simulink model "wcdma_phlayer"  (Simulink 6.0)
settings: Solver=FixedStepDiscrete  SolverMode=SingleTasking  StartTime=0.0  StopTime=0.1  RelTol=1e-3
PreLoadFcn:
  | wcdma_loadinitphlayer;
model workspace: external: M-Code (data not in the file)
undefined symbols (not defined in the file or in its folder): AWGN, Fs, Multipath, slcm, totalBitsDelay, trBlkSetSize, tti
libraries: wcdma_lib x8, dspbuff3 x6, commsink2 x5, dspsnks4 x4, commrandsrc2 x2, commsequence2 x1, dspsigattribs x1, dspsrcs4 x1
CloseFcn:
  | % Clear coding settings
  | clear trBlkSetSize trBlkSize numTrBlks crcSize tti errorCorrMask errorCorr numBitsRF numBitsRM numPhCH posTrCh RMAttribute totalBitsDelay
  | 
  | % Clear antenna settings
  | clear pilotBits overSampling slotFormat sprdFactor scrCode dpchCode numTapsChEst numTapsRRC enableMultipath propConditions
  | 
  | % Clear channel settings
  | clear dopplerFreq snrdB fingerEnables fingerPhases fingerPhasesTicks powerVector fingerPowers
  | 
  | % Clear logging signal
  | clear wcdmaSigsOut
settings Model: Creator=arodrigu  LastModifiedBy=arodrigu  ExtModeAutoUpdateStatusClock=off  ProdHWDeviceType=Specified
settings DataIOCC: LimitDataPoints=off  SaveOutput=off  SaveTime=off  SignalLoggingName=wcdmaSigsOut
settings OptimizationCC: BooleanDataType=off  InlineParams=on
settings DebuggingCC: CheckExecutionContextPreStartOutputMsg=on  CheckExecutionContextRuntimeOutputMsg=on  SolverPrmCheckMsg=none  InheritedTsInSrcMsg=none
settings HardwareCC: ProdHWDeviceType=Specified
settings ModelReferenceCC: UpdateModelReferenceTargets=IfOutOfDate
settings CodeAppCC: MangleLength=5

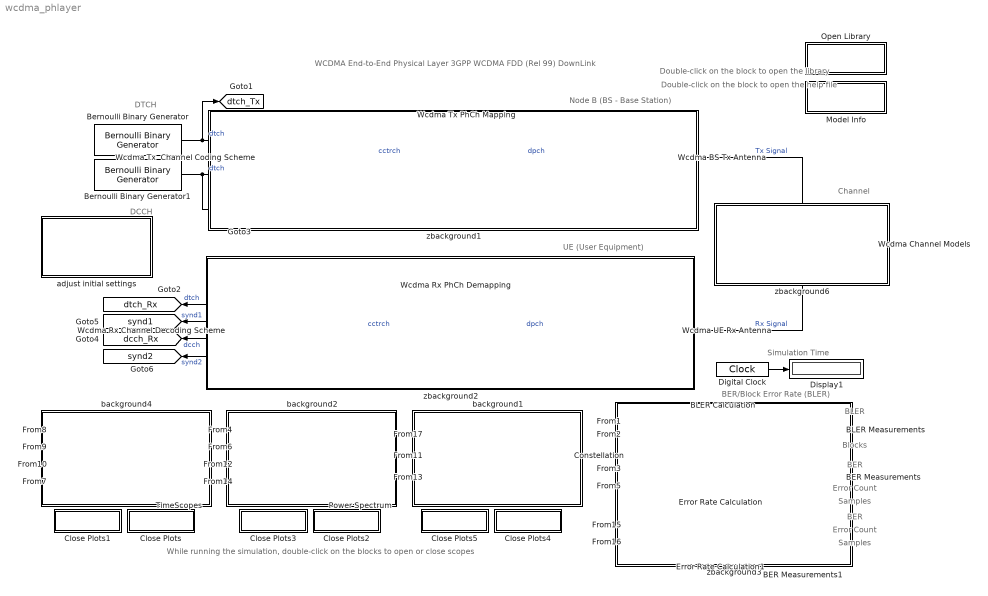
== system wcdma_phlayer ==
  note: DTCH
  note: DCCH
  note: BER
  note: Error Count
  note: Samples
  note: BER/Block Error Rate (BLER)
  note: BLER
  note: Node B (BS - Base Station)
  note: UE (User Equipment)
  note: Channel
  note: WCDMA End-to-End Physical Layer
      | 3GPP WCDMA FDD (Rel 99) DownLink
  note: Blocks
  note: Simulation Time
  note: BER
  note: Error Count
  note: Samples
  note: Double-click on the block
      | to open the help file
  note: While running the simulation, double-click on the blocks to open or close scopes
  note: Double-click on the block
      | to open the library
  BER Measurements : Display
  BER Measurements1 : Display
  BLER Calculation : wcdma_lib/Wcdma Common/BLER Calculation  trBlkSetSize=trBlkSetSize  tti=tti  numBitsDelay=totalBitsDelay
  BLER Measurements : Display
  Bernoulli Binary Generator : commrandsrc2/Bernoulli Binary Generator  P=0.5  seed=[123456]  Ts=(tti(1)*1e-3)/trBlkSetSize(1)  frameBased=on  sampPerFrame=trBlkSetSize(1)  orient=off
  Bernoulli Binary Generator1 : commrandsrc2/Bernoulli Binary Generator  P=0.5  seed=[123456]  Ts=(tti(2)*1e-3)/trBlkSetSize(2)  frameBased=on  sampPerFrame=trBlkSetSize(2)  orient=off
  Close Plots : Subsystem  PropExecContextAcrossSSBoundary=on
      settings: OpenFcn=|
      | ssName = gcs;
      |   set_param([ssName '/TimeScopes/Real Part'],'Open','off');
      |   set_param([ssName '/TimeScopes/Imag Part'],'Open','off');
      |   set_param([ssName '/TimeScopes/Channel Estimates'],'Open','off');
      mask Display: disp('Close Scopes');
  Close Plots1 : Subsystem  PropExecContextAcrossSSBoundary=on
      settings: OpenFcn=|
      | ssName=gcs;
      | set_param([ssName '/TimeScopes/Real Part'],'Open','on');
      |   set_param([ssName '/TimeScopes/Imag Part'],'Open','on');
      |   set_param([ssName '/TimeScopes/Channel Estimates'],'Open','on');
      mask Display: disp('Open Scopes');
  Close Plots2 : Subsystem  PropExecContextAcrossSSBoundary=on
      settings: OpenFcn=|
      | set_param([gcs '/Power Spectrum/Before Spreading Spectrum'],'OpenScopeAtSimStart','off');
      |   set_param([gcs '/Power Spectrum/Before Pulse Shaping'],'OpenScopeAtSimStart','off');
      |   set_param([gcs '/Power Spectrum/Tx Signal'],'OpenScopeAtSimStart','off');
      |   set_param([gcs '/Power Spectrum/Rx Signal'],'OpenScopeAtSimStart','off');
      |   sdspfscope2([],[],[],'ScopeUpdate',[gcs '/Power Spectrum/Before Spreading Spectrum'],'CloseFig');
      |   sdspfscope2([],[],[],'ScopeUpdate',[gcs '/Power Spectrum/Before Pulse Shaping'],'CloseFig');
      |   sdspfscope2([],[],[],'ScopeUpdate',[gcs '/Power Spectrum/Tx Signal'],'CloseFig');
      |   sdspfscope2([],[],[],'ScopeUpdate',[gcs '/Power Spectrum/Rx Signal'],'CloseFig');
      mask Display: disp('Close Scopes');
  Close Plots3 : Subsystem  PropExecContextAcrossSSBoundary=on
      settings: OpenFcn=|
      | set_param([gcs '/Power Spectrum/Before Spreading Spectrum'],'OpenScopeAtSimStart','on');
      |   set_param([gcs '/Power Spectrum/Before Pulse Shaping'],'OpenScopeAtSimStart','on');
      |   set_param([gcs '/Power Spectrum/Tx Signal'],'OpenScopeAtSimStart','on');
      |   set_param([gcs '/Power Spectrum/Rx Signal'],'OpenScopeAtSimStart','on');
      |   sdspfscope2([],[],[],'ScopeUpdate',[gcs '/Power Spectrum/Before Spreading Spectrum'],'OpenFig');
      |   sdspfscope2([],[],[],'ScopeUpdate',[gcs '/Power Spectrum/Before Pulse Shaping'],'OpenFig');
      |   sdspfscope2([],[],[],'ScopeUpdate',[gcs '/Power Spectrum/Tx Signal'],'OpenFig');
      |   sdspfscope2([],[],[],'ScopeUpdate',[gcs '/Power Spectrum/Rx Signal'],'OpenFig');
      mask Display: disp('Open Scopes');
  Close Plots4 : Subsystem  PropExecContextAcrossSSBoundary=on
      settings: OpenFcn=|
      | set_param([bdroot '/Constellation/DPCH_Rx'],'OpenScopeAtSimStart','off');
      | set_param([bdroot '/Constellation/DPCH_Derot'],'OpenScopeAtSimStart','off');
      | set_param([bdroot '/Constellation/DPCH_Comb'],'OpenScopeAtSimStart','off');
      | sdspfscope2([],[],[],'ScopeUpdate',[bdroot '/Constellation/DPCH_Rx'],'CloseFig');
      | sdspfscope2([],[],[],'ScopeUpdate',[bdroot '/Constellation/DPCH_Derot'],'CloseFig');
      | sdspfscope2([],[],[],'ScopeUpdate',[bdroot '/Constellation/DPCH_Comb'],'CloseFig');
      mask Display: disp('Close Scopes');
  Close Plots5 : Subsystem  PropExecContextAcrossSSBoundary=on
      settings: OpenFcn=|
      | sdspfscope2([],[],[],'ScopeUpdate',[bdroot '/Constellation/DPCH_Rx'],'OpenFig');
      | sdspfscope2([],[],[],'ScopeUpdate',[bdroot '/Constellation/DPCH_Derot'],'OpenFig');
      | sdspfscope2([],[],[],'ScopeUpdate',[bdroot '/Constellation/DPCH_Comb'],'OpenFig');
      | set_param([bdroot '/Constellation/DPCH_Rx'],'OpenScopeAtSimStart','on');
      | set_param([bdroot '/Constellation/DPCH_Derot'],'OpenScopeAtSimStart','on');
      | set_param([bdroot '/Constellation/DPCH_Comb'],'OpenScopeAtSimStart','on');
      mask Display: disp('Open Scopes');
  Constellation : Subsystem  TreatAsAtomicUnit=on  PropExecContextAcrossSSBoundary=on
      mask Display: disp('Scatter\nPlot')
  Digital Clock : DigitalClock  SampleTime=0.001
  Display1 : Display
  Error Rate Calculation : commsink2/Error Rate Calculation  N=totalBitsDelay(1)  st_delay=0  cp_mode=Entire frame  subframe=[]  PMode=Port  WsName=ErrorVec  RsMode2=off  stop=off  numErr=100  maxBits=1e6
  Error Rate Calculation1 : commsink2/Error Rate Calculation  N=totalBitsDelay(2)  st_delay=0  cp_mode=Entire frame  subframe=[]  PMode=Port  WsName=ErrorVec  RsMode2=off  stop=off  numErr=100  maxBits=1e6
  Model Info : Subsystem  LoadFcn=slcm LoadBlock;  InitFcn=slcm('UpdateAllCMBlocksInThisModelInit')  PropExecContextAcrossSSBoundary=on  mask(CMBlock){InitialSaveTempField=, InitialBlockCM=none, BlockCM=none, Frame=on, SaveTempField=, DisplayStringWithTags=Info, MaskDisplayString=Info, HorizontalTextAlignment=Center, LeftAlignmentValue=0.5, SourceBlockDiagram=wcdma_phlayer, TagMaxNumber=20, CMTag1=, CMTag2=, CMTag3=, CMTag4=, CMTag5=, CMTag6=, CMTag7=, CMTag8=, CMTag9=, CMTag10=, CMTag11=, CMTag12=, CMTag13=, CMTag14=, CMTag15=, CMTag16=, CMTag17=, CMTag18=, CMTag19=, CMTag20=}
      mask help: This block allows revision control information to be displayed within the model.
      settings: CopyFcn=slcm CopyBlock;  DeleteFcn=slcm Cancel;  PostSaveFcn=slcm('UpdateAllCMBlocksInThisModel')  NameChangeFcn=slcm Rename;  OpenFcn=commdemohelp;
      mask Display: text(str2num(LeftAlignmentValue), 0.5, MaskDisplayString, 'HorizontalAlignment', HorizontalTextAlignment)
  Open Library : Subsystem  PropExecContextAcrossSSBoundary=on
      settings: OpenFcn=open('wcdma_lib.mdl');
      mask Display: disp('WCDMA\nLibrary')
  Power Spectrum : Subsystem  TreatAsAtomicUnit=on  PropExecContextAcrossSSBoundary=on
      mask Display: disp('Power\nSpectrum')
  TimeScopes : Subsystem  TreatAsAtomicUnit=on  PropExecContextAcrossSSBoundary=on
      mask Display: disp('Time\nScopes')
  Wcdma BS Tx Antenna : wcdma_lib/Wcdma BS Transmitter/Wcdma BS Tx Antenna  slotFormat=slotFormat  dpchCode=dpchCode  scrCode=scrCode  powerVector=powerVector  numTapsRRC=numTapsRRC  overSampling=overSampling  checkparams=off
  Wcdma Channel Models : Subsystem  Orientation=down  BlockChoice=Multipath+AWGN  PropExecContextAcrossSSBoundary=on
      settings: AttributesFormatString=%<BlockChoice>  TemplateBlock=wcdma_lib/Wcdma Channel Model/Wcdma Channel Models  MemberBlocks=AWGN,Multipath+AWGN,No Channel
  Wcdma Rx Channel Decoding Scheme : wcdma_lib/Wcdma Multiplexing and Channel Coding/Wcdma Rx Channel Decoding Scheme  Orientation=left  trBlkSetSize=trBlkSetSize  trBlkSize=trBlkSize  tti=tti  crcSize=crcSize  errorCorr=errorCorr  RMAttribute=RMAttribute  posTrCh=posTrCh  numPhCH=numPhCH  slotFormat=slotFormat  checkParams=off
  Wcdma Rx PhCh Demapping : wcdma_lib/Wcdma Multiplexing and Channel Coding/Wcdma Rx PhCh Demapping  Orientation=left  numBitsRF=numBitsRF  numPhCH=numPhCH  slotFormat=slotFormat  checkParams=off
  Wcdma Tx PhCh Mapping : wcdma_lib/Wcdma Multiplexing and Channel Coding/Wcdma Tx PhCh Mapping  numBitsRF=numBitsRF  numPhCH=numPhCH  slotFormat=slotFormat  checkParams=off
  Wcdma Tx  Channel Coding Scheme : wcdma_lib/Wcdma Multiplexing and Channel Coding/Wcdma Tx  Channel Coding Scheme  trBlkSetSize=trBlkSetSize  trBlkSize=trBlkSize  tti=tti  crcSize=crcSize  errorCorr=errorCorr  RMAttribute=RMAttribute  posTrCh=posTrCh  numPhCH=numPhCH  slotFormat=slotFormat  checkParams=off
  Wcdma UE Rx Antenna : wcdma_lib/Wcdma UE Receiver/Wcdma UE Rx Antenna  Orientation=left  slotFormat=slotFormat  dpchCode=dpchCode  scrCode=scrCode  powerVector=powerVector  numTapsRRC=numTapsRRC  overSampling=overSampling  fingerEnables=fingerEnables  fingerPhases=fingerPhases  numTapsChEst=numTapsChEst  checkParams=off
  adjust initial settings : Subsystem  PropExecContextAcrossSSBoundary=on  mask(Wcdma Initial Settings Demo){powerVector=[-5.9 -10 -15 -12 -12], showTrCh=off, measurChannel=12.2 Kbps, trBlkSetSize=[244 100], trBlkSize=[244 100], tti=[20 40], crcSize=[16 12], errorCorr=[2 2], RMAttribute=[256 256], posTrChMask=Fixed, numPhCH=1, slotFormat=11, showAntenna=off, dpchCode=127, scrCode=[63 0], numTapsRRC=96, numTapsChEst=21, overSampling=8, showChModel=off, propConditions=Multipath Profile - Case 6, snrdB=-1, fingerEnables=4, fingerPhases=[0 260e-9 521e-9 781e-9], fingerPowers=[0 -3 -6 -9], speed=250}
      mask prompts: powerVector "Power for [DPCH, P-CPICH, PICH, P-CCPCH, SCH] in dB:"; showTrCh "----------------------------- Show Transport Channel Settings ------------------------------"; measurChannel "DL Measurement channels"; trBlkSetSize "Transport block set size:"; trBlkSize "Transport block size:"; tti "TTI (in ms):"; crcSize "CRC Size {24, 16, 12, 8, 0}:"; errorCorr "Type of error Protection {None=0, Conv 1/2=1, Conv 1/3=2, Turbo=3}:"; RMAttribute "Rate matching attribute:"; posTrChMask "Position of TrCH in radio frame:"; numPhCH "Number of PhCH:"; slotFormat "Slot format (0..16):"; showAntenna "----------------------------- Show Antenna Settings ---------------------------------------"; dpchCode "DPCH Code number (0..Spreading Factor -1):"; scrCode "Scrambling code [Scr Code Grup(0..63) Primary Code(0..7)]:"; numTapsRRC "Number of filter taps for RRC:"; numTapsChEst "Number of coefficients for channel estimation filters:"; overSampling "Oversampling factor:"; showChModel "----------------------------- Show Channel Model Settings -----------------------------"; propConditions "Propagation conditions environments:"; snrdB "SNR (in dB):"; fingerEnables "Number of enable fingers:"; fingerPhases "Relative delay of Rx signals (in s):"; fingerPowers "Average Powers of Rx signals (in dB):"; speed "Speed of Terminal (in Km/h):"
      mask help: Use the following mask to select the different parameters for the simulation.
      mask init:
      | eStr = wcdma_initmaskphlayer(gcb,'init');
      | if(~isempty(eStr.emsg))
      | errordlg(eStr.emsg);
      | end
      | if(~isempty(eStr.emsg_w))
      | disp(eStr.emsg_w);
      | end
      mask Help: eval('commdemohelp;');
      mask StyleString: edit,checkbox,popup(12.2 Kbps|64 Kbps|144 Kbps|384 Kbps|User Defined),edit,edit,edit,edit,edit,edit,popup(Fixed|Flexible),popup(1|2|3),popup(0|1|2|3|4|5|6|7|8|9|10|11|12|13|14|15|16),checkbox,edit,edit,edit,edit,popup(2|4|6|8|10|12|14|16),checkbox,popup(No Channel|Static - AWGN|Multipath Profile - Case 1|Multipath Profile - Case 2|Multipath Profile - Case 3|Multipath Profile - Case 4|Multipath Profile - Case 5|Multipath Profile - Case 6|User Defined),edit,popup(1|2|3|4),edit,edit,edit
      mask CallbackString: |wcdma_initmaskphlayer(gcb,'cbShowTrCh');|wcdma_initmaskphlayer(gcb,'cbMeasurChannel');||||||||||wcdma_initmaskphlayer(gcb,'cbShowAntenna');||||||wcdma_initmaskphlayer(gcb,'cbShowChModel');|wcdma_initmaskphlayer(gcb,'cbPropConditions');|||||
      mask Display: disp('Wcdma Demo:\nInitial Settings');
  background1 : Subsystem  PropExecContextAcrossSSBoundary=on
      mask Display: disp('')
  background2 : Subsystem  PropExecContextAcrossSSBoundary=on
      mask Display: disp('')
  background4 : Subsystem  PropExecContextAcrossSSBoundary=on
      mask Display: disp('')
  zbackground1 : Subsystem  Priority=0  PropExecContextAcrossSSBoundary=on
      mask Display: disp('')
  zbackground2 : Subsystem  PropExecContextAcrossSSBoundary=on
      mask Display: disp('')
  zbackground3 : Subsystem  PropExecContextAcrossSSBoundary=on
      mask Display: disp('')
  zbackground6 : Subsystem  PropExecContextAcrossSSBoundary=on
      mask Display: disp('');
  tag scope: dcch_Rx=global, dcch_Tx=global, dtch_Rx=global, dtch_Tx=global, synd1=global, synd2=global
  wires:
  Bernoulli Binary Generator/1 -> Wcdma Tx  Channel Coding Scheme/1, [dtch_Tx]  "dtch"
  [dtch_Tx] -> Error Rate Calculation/1
  [dtch_Rx] -> Error Rate Calculation/2
  Wcdma Rx Channel Decoding Scheme/1 -> [dtch_Rx]  "dtch"
  Wcdma Rx Channel Decoding Scheme/3 -> [dcch_Rx]  "dcch"
  Wcdma Rx PhCh Demapping/1 -> Wcdma Rx Channel Decoding Scheme/1  "cctrch"
  Wcdma UE Rx Antenna/1 -> Wcdma Rx PhCh Demapping/1  "dpch"
  BLER Calculation/1 -> BLER Measurements/1
  Wcdma Rx Channel Decoding Scheme/2 -> [synd1]  "synd1"
  Wcdma Rx Channel Decoding Scheme/4 -> [synd2]  "synd2"
  [synd1] -> BLER Calculation/1
  [synd2] -> BLER Calculation/2
  Digital Clock/1 -> Display1/1
  Wcdma Tx  Channel Coding Scheme/1 -> Wcdma Tx PhCh Mapping/1  "cctrch"
  Wcdma BS Tx Antenna/1 -> Wcdma Channel Models/1(ChIn)  "Tx Signal"
  Wcdma Channel Models/1(ChOut) -> Wcdma UE Rx Antenna/1  "Rx Signal"
  Bernoulli Binary Generator1/1 -> Wcdma Tx  Channel Coding Scheme/2, [dcch_Tx]  "dtch"
  Wcdma Tx PhCh Mapping/1 -> Wcdma BS Tx Antenna/1  "dpch"
  [dcch_Tx] -> Error Rate Calculation1/1
  [dcch_Rx] -> Error Rate Calculation1/2
  [DPCH_Tx] -> TimeScopes/1(In1)
  [DPCH_Tx_sprd] -> TimeScopes/2(In2)
  [DPCH_Tx_all] -> TimeScopes/3(In3)
  [chEst] -> TimeScopes/4(In5)
  [DPCH_Tx] -> Power Spectrum/1(In1)
  [DPCH_Tx_all] -> Power Spectrum/2(In3)
  [ToChannel] -> Power Spectrum/3(In4)
  [RxSignal] -> Power Spectrum/4(In6)
  Error Rate Calculation/1 -> BER Measurements/1
  Error Rate Calculation1/1 -> BER Measurements1/1
  [DPCH_Rx] -> Constellation/1(In1)
  [DPCH_Derot] -> Constellation/2(In2)
  [DPCH_Comb] -> Constellation/3(In3)

== system wcdma_phlayer/Close Plots ==

== system wcdma_phlayer/Close Plots1 ==

== system wcdma_phlayer/Close Plots2 ==

== system wcdma_phlayer/Close Plots3 ==

== system wcdma_phlayer/Close Plots4 ==

== system wcdma_phlayer/Close Plots5 ==

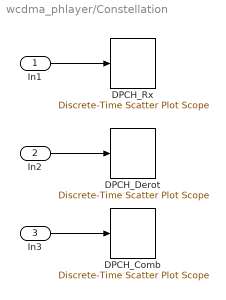
== system wcdma_phlayer/Constellation ==
  In1 : Inport  LatchInput=off
  In2 : Inport  Port=2  LatchInput=off
  In3 : Inport  Port=3  LatchInput=off
  DPCH_Comb : commsink2/Discrete-Time Scatter Plot Scope  Tag=ScatterPlot  sampPerSymb=1  offsetEye=0  numTraces=70  numNewFrames=20  LineMarkers=.  LineColors=[1 0 1]  fading=on  render=off  AxisGrid=on  xMin=-2.7  xMax=2.7  yMin=-2.7  yMax=2.7  inphaseLabel=In-phase Amplitude  quadratureLabel=Quadrature Amplitude  openScopeAtSimStart=off  FrameNumber=off  FigPos=[685 314 327 327]  figTitle=Scatter Plot  numLinesMax=50  block_type_=scatter
  DPCH_Derot : commsink2/Discrete-Time Scatter Plot Scope  Tag=ScatterPlot  sampPerSymb=1  offsetEye=0  numTraces=30  numNewFrames=5  LineMarkers=.  LineColors=b  fading=on  render=off  AxisGrid=on  xMin=-0.364657245618191  xMax=0.344086050451824  yMin=-0.372605059946187  yMax=0.336138236123828  inphaseLabel=In-phase Amplitude  quadratureLabel=Quadrature Amplitude  openScopeAtSimStart=off  FrameNumber=off  FigPos=[344 313 328 328]  figTitle=Scatter Plot  numLinesMax=50  block_type_=scatter
  DPCH_Rx : commsink2/Discrete-Time Scatter Plot Scope  Tag=ScatterPlot  sampPerSymb=1  offsetEye=0  numTraces=30  numNewFrames=6  LineMarkers=.  LineColors=[1 0 0]  fading=on  render=off  AxisGrid=on  xMin=-0.857650806774146  xMax=0.765534044638798  yMin=-0.74851489261803  yMax=0.874669958794914  inphaseLabel=In-phase Amplitude  quadratureLabel=Quadrature Amplitude  openScopeAtSimStart=off  FrameNumber=off  FigPos=[12 320 320 320]  figTitle=Scatter Plot  numLinesMax=50  block_type_=scatter
  wires:
  In1/1 -> DPCH_Rx/1
  In2/1 -> DPCH_Derot/1
  In3/1 -> DPCH_Comb/1

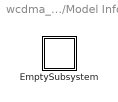
== system wcdma_phlayer/Model Info ==
  EmptySubsystem : Subsystem  PropExecContextAcrossSSBoundary=on

== system wcdma_phlayer/Open Library ==
  note: This subsystem is intentionally left empty

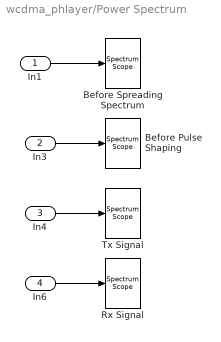
== system wcdma_phlayer/Power Spectrum ==
  In1 : Inport  LatchInput=off
  In3 : Inport  Port=2  LatchInput=off
  In4 : Inport  Port=3  LatchInput=off
  In6 : Inport  Port=4  LatchInput=off
  Before Pulse Shaping : dspsnks4/Spectrum Scope  ScopeProperties=on  Domain=Frequency  HorizSpan=1  UseBuffer=on  BufferSize=256  Overlap=0  inpFftLenInherit=off  FFTlength=128  numAvg=20  DisplayProperties=off  AxisGrid=on  Memory=off  FrameNumber=off  AxisLegend=off  AxisZoom=off  OpenScopeAtSimStart=off  OpenScopeImmediately=off  FigPos=[358 496 308 199]  AxisProperties=off  XUnits=Hertz  XRange=[-Fs/2...Fs/2]  InheritXIncr=on  XIncr=1.0  XLabel=Samples  YUnits=dB  YLabel=Magnitude, dB  LineProperties=off  LineColors=[1 0 0]
      settings: YMin=-20  YMax=20
  Before Spreading Spectrum : dspsnks4/Spectrum Scope  ScopeProperties=on  Domain=Frequency  HorizSpan=1  UseBuffer=on  BufferSize=64  Overlap=0  inpFftLenInherit=off  FFTlength=128  numAvg=2  DisplayProperties=off  AxisGrid=on  Memory=off  FrameNumber=off  AxisLegend=off  AxisZoom=off  OpenScopeAtSimStart=off  OpenScopeImmediately=off  FigPos=[29 496 308 199]  AxisProperties=off  XUnits=Hertz  XRange=[-Fs/2...Fs/2]  InheritXIncr=on  XIncr=1.0  XLabel=Samples  YUnits=Magnitude  YLabel=Magnitude, dB  LineProperties=off  LineColors=[1 0 0]
      settings: YMin=-0.913387640631292  YMax=19.2304598955481
  Rx Signal : dspsnks4/Spectrum Scope  ScopeProperties=on  Domain=Frequency  HorizSpan=1  UseBuffer=on  BufferSize=2048  Overlap=0  inpFftLenInherit=off  FFTlength=128  numAvg=100  DisplayProperties=off  AxisGrid=on  Memory=off  FrameNumber=off  AxisLegend=off  AxisZoom=off  OpenScopeAtSimStart=off  OpenScopeImmediately=off  FigPos=[289 234 381 201]  AxisProperties=off  XUnits=Hertz  XRange=[-Fs/2...Fs/2]  InheritXIncr=on  XIncr=1.0  XLabel=Samples  YUnits=dB  YLabel=Magnitude, dB  LineProperties=off  LineColors=[1 0 0]
      settings: YMin=10.012094494741  YMax=17.9084191472902
  Tx Signal : dspsnks4/Spectrum Scope  ScopeProperties=on  Domain=Frequency  HorizSpan=1  UseBuffer=on  BufferSize=2048  Overlap=0  inpFftLenInherit=off  FFTlength=128  numAvg=100  DisplayProperties=off  AxisGrid=on  Memory=off  FrameNumber=off  AxisLegend=off  AxisZoom=off  OpenScopeAtSimStart=off  OpenScopeImmediately=off  FigPos=[695 496 308 198]  AxisProperties=off  XUnits=Hertz  XRange=[-Fs/2...Fs/2]  InheritXIncr=on  XIncr=1.0  XLabel=Samples  YUnits=dB  YLabel=Magnitude, dB  LineProperties=off  LineColors=[1 0 0]
      settings: YMin=-50  YMax=20
  wires:
  In6/1 -> Rx Signal/1
  In4/1 -> Tx Signal/1
  In3/1 -> Before Pulse Shaping/1
  In1/1 -> Before Spreading Spectrum/1

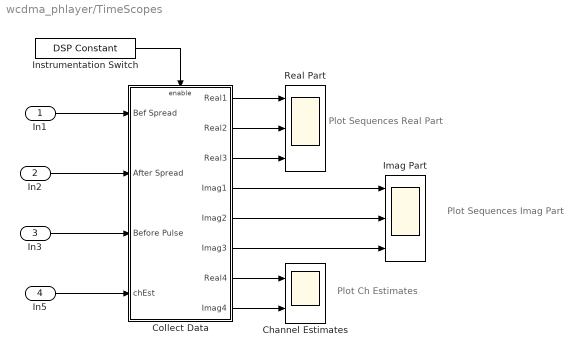
== system wcdma_phlayer/TimeScopes ==
  note: Plot Sequences
      | Real Part
  note: Plot Sequences
      | Imag Part
  note: Plot
      | Ch Estimates
  In1 : Inport  LatchInput=off
  In2 : Inport  Port=2  LatchInput=off
  In3 : Inport  Port=3  LatchInput=off
  In5 : Inport  Port=4  LatchInput=off
  Channel Estimates : Scope  NumInputPorts=2
      settings: TimeRange=0.1  YMin=-0.15~-0.35  YMax=0.5~0.3  SaveName=ScopeData4  DataFormat=Structure
  Collect Data : Subsystem  TreatAsAtomicUnit=on  PropExecContextAcrossSSBoundary=on
  Imag Part : Scope  NumInputPorts=3
      settings: TimeRange=0.0001500000000000008  YMin=-0.5~-1.5~-1.5  YMax=1.5~1.5~1.5  SaveName=ScopeData5  DataFormat=Structure  MaxDataPoints=512
  Instrumentation Switch : dspsrcs4/DSP Constant  Value=1  SampleMode=Discrete  discreteOutput=Sample-based  continuousOutput=Sample-based  sampTime=1/15e3  framePeriod=1/15e3  dataType=Inherit from 'Constant value'  isSigned=on  wordLen=16  udDataType=sfix(16)  fracBitsMode=Best precision  numFracBits=15  InterpretAs1D=off  Ts=1/15e3  FramebasedOutput=off
  Real Part : Scope  NumInputPorts=3
      settings: TimeRange=0.0001500000000000008  YMin=-0.5~-1.5~-1.5  YMax=1.5~1.5~1.5  SaveName=ScopeData6  DataFormat=Structure  MaxDataPoints=512
  wires:
  Collect Data/8(Imag4) -> Channel Estimates/2
  Collect Data/7(Real4) -> Channel Estimates/1
  Instrumentation Switch/1 -> Collect Data/Enable
  Collect Data/6(Imag3) -> Imag Part/3
  Collect Data/5(Imag2) -> Imag Part/2
  Collect Data/4(Imag1) -> Imag Part/1
  Collect Data/3(Real3) -> Real Part/3
  Collect Data/2(Real2) -> Real Part/2
  Collect Data/1(Real1) -> Real Part/1
  In1/1 -> Collect Data/1(Bef Spread)
  In2/1 -> Collect Data/2(After Spread)
  In3/1 -> Collect Data/3(Before Pulse)
  In5/1 -> Collect Data/4(chEst)

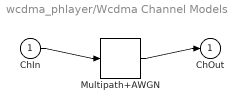
== system wcdma_phlayer/Wcdma Channel Models ==
  ChIn : Inport  LatchInput=off
  Multipath+AWGN : wcdma_lib/Wcdma Channel Model/Multipath+AWGN
  ChOut : Outport
  wires:
  ChIn/1 -> Multipath+AWGN/1
  Multipath+AWGN/1 -> ChOut/1

== system wcdma_phlayer/adjust initial settings ==

== system wcdma_phlayer/background1 ==

== system wcdma_phlayer/background2 ==

== system wcdma_phlayer/background4 ==

== system wcdma_phlayer/zbackground1 ==

== system wcdma_phlayer/zbackground2 ==

== system wcdma_phlayer/zbackground3 ==

== system wcdma_phlayer/zbackground6 ==

== system wcdma_phlayer/Model Info/EmptySubsystem ==

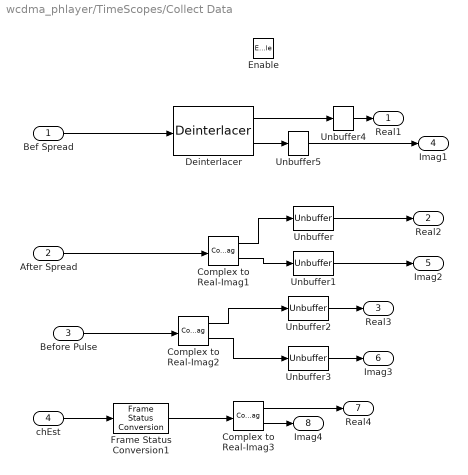
== system wcdma_phlayer/TimeScopes/Collect Data ==
  Bef Spread : Inport  LatchInput=off
  After Spread : Inport  Port=2  LatchInput=off
  Before Pulse : Inport  Port=3  LatchInput=off
  chEst : Inport  Port=4  LatchInput=off
  Enable : EnablePort
  Complex to Real-Imag1 : ComplexToRealImag
  Complex to Real-Imag2 : ComplexToRealImag
  Complex to Real-Imag3 : ComplexToRealImag
  Deinterlacer : commsequence2/Deinterlacer
  Frame Status Conversion1 : dspsigattribs/Frame Status Conversion  growRefPort=off  outframe=Sample-based
  Unbuffer{,1..5} (6 alike) : dspbuff3/Unbuffer  ic=0
  Real1 : Outport
  Real2 : Outport  Port=2
  Real3 : Outport  Port=3
  Imag1 : Outport  Port=4
  Imag2 : Outport  Port=5
  Imag3 : Outport  Port=6
  Real4 : Outport  Port=7
  Imag4 : Outport  Port=8
  wires:
  Frame Status Conversion1/1 -> Complex to Real-Imag3/1
  Unbuffer5/1 -> Imag1/1
  Unbuffer4/1 -> Real1/1
  Deinterlacer/2 -> Unbuffer5/1
  Deinterlacer/1 -> Unbuffer4/1
  chEst/1 -> Frame Status Conversion1/1
  Complex to Real-Imag3/2 -> Imag4/1
  Complex to Real-Imag3/1 -> Real4/1
  Unbuffer3/1 -> Imag3/1
  Unbuffer2/1 -> Real3/1
  Before Pulse/1 -> Complex to Real-Imag2/1
  Complex to Real-Imag2/1 -> Unbuffer2/1
  Complex to Real-Imag2/2 -> Unbuffer3/1
  Complex to Real-Imag1/1 -> Unbuffer/1
  Unbuffer1/1 -> Imag2/1
  Unbuffer/1 -> Real2/1
  Complex to Real-Imag1/2 -> Unbuffer1/1
  After Spread/1 -> Complex to Real-Imag1/1
  Bef Spread/1 -> Deinterlacer/1
